simulink model "Lab2_3"  (Simulink 7.3)
settings: Solver=ode45  StartTime=0.0  StopTime=1.0  RelTol=1e-3
libraries: simulink x1
settings Model: Creator=Seva  LastModifiedBy=Seva

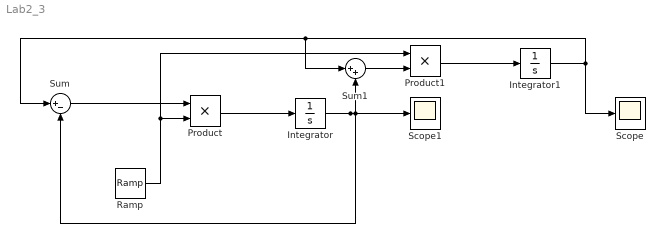
== system Lab2_3 ==
  Integrator : Integrator  InitialCondition=1
  Integrator1 : Integrator  InitialCondition=1
  Product : Product  OutDataType=fixdt(1, 16)  OutScaling=2^0  RndMeth=Zero
  Product1 : Product  OutDataType=fixdt(1, 16)  OutScaling=2^0  RndMeth=Zero
  Ramp : simulink/Sources/Ramp  SystemSampleTime=-1  slope=1  start=0  X0=0
  Scope : Scope
  Scope1 : Scope
  Sum : Sum  Inputs=|+-  OutDataType=fixdt(1, 16)  OutScaling=2^0
  Sum1 : Sum  Inputs=|++  OutDataType=fixdt(1, 16)  OutScaling=2^0
  wires:
  Sum/1 -> Product/1
  Ramp/1 -> Product/2, Product1/1
  Product/1 -> Integrator/1
  Integrator/1 -> Sum/2, Sum1/2, Scope1/1
  Sum1/1 -> Product1/2
  Product1/1 -> Integrator1/1
  Integrator1/1 -> Sum1/1, Sum/1, Scope/1
